simulink model "gm_hybrid_lht"  (R2019b)
settings: Solver=FixedStepDiscrete  StartTime=0.0  StopTime=inf  FixedStep=1/120e6  RelTol=1e-3
undefined symbols (not defined in the file or in its folder): bt, height, nTheta, width
libraries: hdlsllib x612, simulink x494, hdlmdlgenlib x7, dspsrcs4 x1
(part 2 of 17)

== system gm_hybrid_lht/Hybrid LHT/Hybrid LHT Kernel/Extract Active Votes ==
  note: Check the indices to ensure they are in the correct limits
  Theta : Inport  OutDataTypeStr=uint8  PortDimensions=1  SampleTime=8.33333333333333e-09
  Add : Sum  AccumDataTypeStr=fixdt(1, 10, 0)  OutDataTypeStr=fixdt(1, 10, 0)  SampleTime=8.33333333333333e-09
  Add1 : Sum  Inputs=+-  AccumDataTypeStr=fixdt(1, 12, 0)  OutDataTypeStr=fixdt(1, 12, 0)  SampleTime=8.33333333333333e-09
  Add2 : Sum  Inputs=+-  AccumDataTypeStr=fixdt(1, 9, 0)  OutDataTypeStr=fixdt(1, 9, 0)  SampleTime=8.33333333333333e-09
  Add3 : Sum  AccumDataTypeStr=fixdt(1, 11, 0)  OutDataTypeStr=fixdt(1, 11, 0)  SampleTime=8.33333333333333e-09
  Add4 : Sum  Inputs=+-  AccumDataTypeStr=uint8  OutDataTypeStr=uint8  SampleTime=8.33333333333333e-09
  Constant : Constant  Value=[-30 -29 -28 -27 -26 -25 -24 -23 -22 -21 -20 -19 -18 -17 -16 -15 -14 -13 -12 -11 -10 -9 -8 -7 -6 -5 -4 -3 -2 -1 0 1 2 3 4 5 6 7 8 9 10 11 12 13 14 15 16 17 18 19 20 21 22 23 24 25 26 27 28 29]  VectorParams1D=off  OutDataTypeStr=fixdt(1, 6, 0)  SampleTime=-1
  Data Type Conversion : DataTypeConversion  OutDataTypeStr=uint8  SampleTime=8.33333333333333e-09
  Data Type Conversion1 : DataTypeConversion  OutDataTypeStr=uint8  SampleTime=8.33333333333333e-09
  Gain1 : Product  Inputs=**  OutDataTypeStr=uint8  SampleTime=8.33333333333333e-09
  Gain1_const : Constant  Value=60  OutDataTypeStr=uint8  SampleTime=-1
  GetShift : Subsystem
  High : Constant  Value=59  OutDataTypeStr=uint8  SampleTime=-1
  High1 : Constant  Value=59  OutDataTypeStr=uint8  SampleTime=-1
  Low : Constant  Value=0  OutDataTypeStr=fixdt(0, 1, 0)  SampleTime=-1
  Multiport Switch2 : MultiPortSwitch  DataPortOrder=Zero-based contiguous  Inputs=2  DiagnosticForDefault=None  zeroidx=on  OutDataTypeStr=fixdt(1, 11, 0)  SampleTime=8.33333333333333e-09
  Multiport Switch3 : MultiPortSwitch  DataPortOrder=Zero-based contiguous  Inputs=2  DiagnosticForDefault=None  zeroidx=on  OutDataTypeStr=fixdt(1, 12, 0)  SampleTime=8.33333333333333e-09
  PipelineRegister : Delay  DelayLength=double(1)  InitialCondition=0  SampleTime=8.33333333333333e-09
  Relational : RelationalOperator  Operator=<  OutDataTypeStr=boolean  SampleTime=8.33333333333333e-09  RndMeth=Nearest
  Relational1 : RelationalOperator  Operator=>  OutDataTypeStr=boolean  SampleTime=8.33333333333333e-09  RndMeth=Nearest
  Selector4 : Selector  NumberOfDimensions=2  IndexMode=Zero-based  SampleTime=8.33333333333333e-09  IndexOptions=Index vector (dialog),Index vector (dialog)  Indices=double(0),double([59 58 57 56 55 54 53 52 51 50 49 48 47 46 45 44 43 42 41 40 39 38 37 36 35 34 33 32 31 30 29 28 27 26 25 24 23 22 21 20 19 18 17 16 15 14 13 12 11 10 9 8 7 6 5 4 3 2 1 0])  OutputSizes=double(1),double(1)
  delayMatch : Delay  DelayLength=double(1)  InitialCondition=0  SampleTime=8.33333333333333e-09
  nTheta : Constant  Value=60  OutDataTypeStr=uint8  SampleTime=-1
  Index : Outport  VectorParamsAs1DForOutWhenUnconnected=off
  wires:
  delayMatch/1 -> Add2/1
  Add/1 -> Relational/1, Multiport Switch2/2, Add3/1
  Add1/1 -> Multiport Switch3/3
  Add2/1 -> Add/1
  Add3/1 -> Multiport Switch2/3
  Add4/1 -> Selector4/1
  Constant/1 -> Add/2
  Data Type Conversion/1 -> Data Type Conversion1/1
  Data Type Conversion1/1 -> Add4/2
  PipelineRegister/1 -> Add2/2
  GetShift/1(Shift) -> Gain1/2
  High/1 -> Relational1/2
  High1/1 -> Add4/1
  Low/1 -> Relational/2
  Multiport Switch2/1 -> Relational1/1, Multiport Switch3/2, Add1/1
  Multiport Switch3/1 -> Data Type Conversion/1
  Relational/1 -> Multiport Switch2/1
  Relational1/1 -> Multiport Switch3/1
  Selector4/1 -> Index/1
  nTheta/1 -> Add3/2, Add1/2
  Gain1_const/1 -> Gain1/1
  Theta/1 -> delayMatch/1, GetShift/1(Theta)
  Gain1/1 -> PipelineRegister/1

== system gm_hybrid_lht/Hybrid LHT/Hybrid LHT Kernel/Gradient Kernel System ==
  Edge : Inport  OutDataTypeStr=fixdt(0, 1, 0)  PortDimensions=1  SampleTime=8.33333333333333e-09
  X : Inport  Port=2  OutDataTypeStr=fixdt(1, 10, 0)  PortDimensions=1  SampleTime=8.33333333333333e-09
  Y : Inport  Port=3  OutDataTypeStr=fixdt(1, 10, 0)  PortDimensions=1  SampleTime=8.33333333333333e-09
  Theta : Inport  Port=4  OutDataTypeStr=uint8  PortDimensions=1  SampleTime=8.33333333333333e-09
  Get Index and Fix Limits : Subsystem
  Hough Kernel : Subsystem
  vEdge : Outport  VectorParamsAs1DForOutWhenUnconnected=off
  Rho : Outport  Port=2  VectorParamsAs1DForOutWhenUnconnected=off
  Shift : Outport  Port=3  VectorParamsAs1DForOutWhenUnconnected=off
  wires:
  Get Index and Fix Limits/1(Index) -> Hough Kernel/4(Index)
  Get Index and Fix Limits/2(Shift) -> Shift/1
  Hough Kernel/1(vEdge) -> vEdge/1
  Hough Kernel/2(Rho) -> Rho/1
  Edge/1 -> Hough Kernel/1(Edge)
  X/1 -> Hough Kernel/2(X)
  Y/1 -> Hough Kernel/3(Y)
  Theta/1 -> Get Index and Fix Limits/1(Theta)

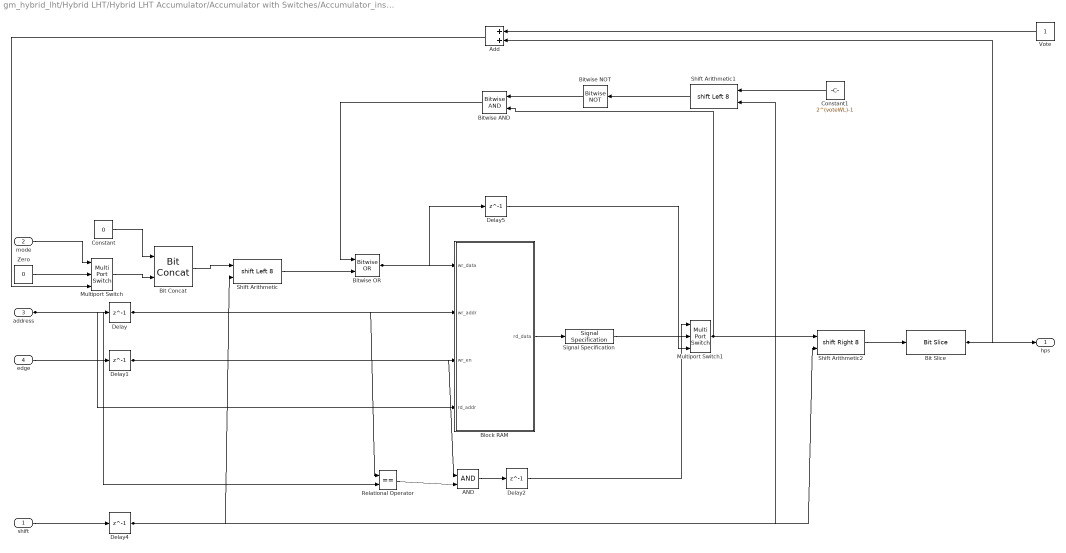
== system gm_hybrid_lht/Hybrid LHT/Hybrid LHT Accumulator/Accumulator with Switches/Accumulator_instance1 ==
  shift : Inport  OutDataTypeStr=fixdt(0, 6, 0)  PortDimensions=1  SampleTime=8.33333333333333e-09
  mode : Inport  Port=2  OutDataTypeStr=boolean  PortDimensions=1  SampleTime=8.33333333333333e-09
  address : Inport  Port=3  OutDataTypeStr=fixdt(0, 11, 0)  PortDimensions=1  SampleTime=8.33333333333333e-09
  edge : Inport  Port=4  OutDataTypeStr=boolean  PortDimensions=1  SampleTime=8.33333333333333e-09
  AND : Logic  IconShape=distinctive  AllPortsSameDT=off  OutDataTypeStr=boolean
  Add : Sum  OutDataTypeStr=fixdt(0, ceil(log2(maxRho*2)), 0)
  Bit Concat : hdlsllib/Logic and Bit Operations/Bit Concat  numInputs=2
      settings: SourceProductName=Simulink
  Bit Slice : hdlsllib/Logic and Bit Operations/Bit Slice  lidx=voteWL-1  ridx=0
  Bitwise AND : simulink/Logic and Bit Operations/Bitwise Operator  logicop=AND  UseBitMask=off  NumInputPorts=2  BitMask=bin2dec('11011001')  BitMaskRealWorld=Stored Integer
  Bitwise NOT : simulink/Logic and Bit Operations/Bitwise Operator  logicop=NOT  UseBitMask=off  BitMask=bin2dec('11011001')  BitMaskRealWorld=Stored Integer
  Bitwise OR : simulink/Logic and Bit Operations/Bitwise Operator  logicop=OR  UseBitMask=off  NumInputPorts=2  BitMask=bin2dec('11011001')  BitMaskRealWorld=Stored Integer
  Block RAM : Subsystem
  Constant : Constant  Value=0  OutDataTypeStr=fixdt(0, 36-voteWL, 0)  SampleTime=-1
  Constant1 : Constant  Value=2^(voteWL)-1  OutDataTypeStr=fixdt(0, 36, 0)  SampleTime=-1
  Delay{,1..2,4..5} (5 alike) : Delay  DelayLength=1
  Multiport Switch : MultiPortSwitch  DataPortOrder=Zero-based contiguous  Inputs=2  zeroidx=on
  Multiport Switch1 : MultiPortSwitch  DataPortOrder=Zero-based contiguous  Inputs=2  zeroidx=on
  Relational Operator : RelationalOperator  Operator===  OutDataTypeStr=boolean  RndMeth=Simplest
  Shift Arithmetic : ArithShift  BitShiftNumberSource=Input port  BitShiftNumber=8  BitShiftDirection=Left  DiagnosticForOORShift=Error
      settings: InputPortMap=u0,p1
  Shift Arithmetic1 : ArithShift  BitShiftNumberSource=Input port  BitShiftNumber=8  BitShiftDirection=Left  DiagnosticForOORShift=Error
      settings: InputPortMap=u0,p1
  Shift Arithmetic2 : ArithShift  BitShiftNumberSource=Input port  BitShiftNumber=8  BitShiftDirection=Right  DiagnosticForOORShift=Error
      settings: InputPortMap=u0,p1
  Signal Specification : SignalSpecification  OutDataTypeStr=fixdt(0, 36, 0)
  Vote : Constant  OutDataTypeStr=fixdt(0,1,0)  SampleTime=-1
  Zero : Constant  Value=0  OutDataTypeStr=fixdt(0,1,0)  SampleTime=-1
  hps : Outport
  wires:
  Zero/1 -> Multiport Switch/2
  Vote/1 -> Add/1
  Shift Arithmetic1/1 -> Bitwise NOT/1
  Relational Operator/1 -> AND/2
  Delay4/1 -> Shift Arithmetic1/2, Shift Arithmetic/2, Shift Arithmetic2/2
  Delay2/1 -> Multiport Switch1/1
  Delay1/1 -> AND/1, Block RAM/3(wr_en)
  Delay/1 -> Relational Operator/1, Block RAM/2(wr_addr)
  Constant1/1 -> Shift Arithmetic1/1
  Constant/1 -> Bit Concat/1
  Bitwise NOT/1 -> Bitwise AND/1
  Bit Slice/1 -> hps/1, Add/2
  AND/1 -> Delay2/1
  shift/1 -> Delay4/1
  mode/1 -> Multiport Switch/1
  address/1 -> Relational Operator/2, Delay/1, Block RAM/4(rd_addr)
  edge/1 -> Delay1/1
  Delay5/1 -> Multiport Switch1/3
  Shift Arithmetic/1 -> Bitwise OR/2
  Bit Concat/1 -> Shift Arithmetic/1
  Multiport Switch/1 -> Bit Concat/2
  Add/1 -> Multiport Switch/3
  Shift Arithmetic2/1 -> Bit Slice/1
  Bitwise AND/1 -> Bitwise OR/1
  Bitwise OR/1 -> Delay5/1, Block RAM/1(wr_data)
  Signal Specification/1 -> Multiport Switch1/2
  Multiport Switch1/1 -> Bitwise AND/2, Shift Arithmetic2/1
  Block RAM/1(rd_data) -> Signal Specification/1

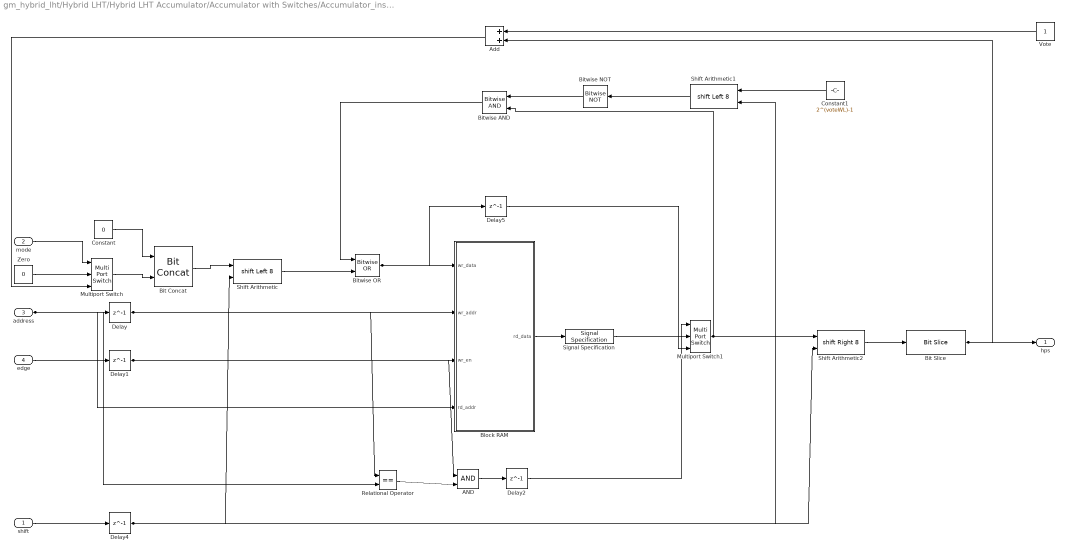
== system gm_hybrid_lht/Hybrid LHT/Hybrid LHT Accumulator/Accumulator with Switches/Accumulator_instance10 ==
  shift : Inport  OutDataTypeStr=fixdt(0, 6, 0)  PortDimensions=1  SampleTime=8.33333333333333e-09
  mode : Inport  Port=2  OutDataTypeStr=boolean  PortDimensions=1  SampleTime=8.33333333333333e-09
  address : Inport  Port=3  OutDataTypeStr=fixdt(0, 11, 0)  PortDimensions=1  SampleTime=8.33333333333333e-09
  edge : Inport  Port=4  OutDataTypeStr=boolean  PortDimensions=1  SampleTime=8.33333333333333e-09
  AND : Logic  IconShape=distinctive  AllPortsSameDT=off  OutDataTypeStr=boolean
  Add : Sum  OutDataTypeStr=fixdt(0, ceil(log2(maxRho*2)), 0)
  Bit Concat : hdlsllib/Logic and Bit Operations/Bit Concat  numInputs=2
      settings: SourceProductName=Simulink
  Bit Slice : hdlsllib/Logic and Bit Operations/Bit Slice  lidx=voteWL-1  ridx=0
  Bitwise AND : simulink/Logic and Bit Operations/Bitwise Operator  logicop=AND  UseBitMask=off  NumInputPorts=2  BitMask=bin2dec('11011001')  BitMaskRealWorld=Stored Integer
  Bitwise NOT : simulink/Logic and Bit Operations/Bitwise Operator  logicop=NOT  UseBitMask=off  BitMask=bin2dec('11011001')  BitMaskRealWorld=Stored Integer
  Bitwise OR : simulink/Logic and Bit Operations/Bitwise Operator  logicop=OR  UseBitMask=off  NumInputPorts=2  BitMask=bin2dec('11011001')  BitMaskRealWorld=Stored Integer
  Block RAM : Subsystem
  Constant : Constant  Value=0  OutDataTypeStr=fixdt(0, 36-voteWL, 0)  SampleTime=-1
  Constant1 : Constant  Value=2^(voteWL)-1  OutDataTypeStr=fixdt(0, 36, 0)  SampleTime=-1
  Delay{,1..2,4..5} (5 alike) : Delay  DelayLength=1
  Multiport Switch : MultiPortSwitch  DataPortOrder=Zero-based contiguous  Inputs=2  zeroidx=on
  Multiport Switch1 : MultiPortSwitch  DataPortOrder=Zero-based contiguous  Inputs=2  zeroidx=on
  Relational Operator : RelationalOperator  Operator===  OutDataTypeStr=boolean  RndMeth=Simplest
  Shift Arithmetic : ArithShift  BitShiftNumberSource=Input port  BitShiftNumber=8  BitShiftDirection=Left  DiagnosticForOORShift=Error
      settings: InputPortMap=u0,p1
  Shift Arithmetic1 : ArithShift  BitShiftNumberSource=Input port  BitShiftNumber=8  BitShiftDirection=Left  DiagnosticForOORShift=Error
      settings: InputPortMap=u0,p1
  Shift Arithmetic2 : ArithShift  BitShiftNumberSource=Input port  BitShiftNumber=8  BitShiftDirection=Right  DiagnosticForOORShift=Error
      settings: InputPortMap=u0,p1
  Signal Specification : SignalSpecification  OutDataTypeStr=fixdt(0, 36, 0)
  Vote : Constant  OutDataTypeStr=fixdt(0,1,0)  SampleTime=-1
  Zero : Constant  Value=0  OutDataTypeStr=fixdt(0,1,0)  SampleTime=-1
  hps : Outport
  wires:
  Block RAM/1(rd_data) -> Signal Specification/1
  Multiport Switch1/1 -> Shift Arithmetic2/1, Bitwise AND/2
  Signal Specification/1 -> Multiport Switch1/2
  Bitwise OR/1 -> Block RAM/1(wr_data), Delay5/1
  Bitwise AND/1 -> Bitwise OR/1
  Shift Arithmetic2/1 -> Bit Slice/1
  Add/1 -> Multiport Switch/3
  Multiport Switch/1 -> Bit Concat/2
  Bit Concat/1 -> Shift Arithmetic/1
  Shift Arithmetic/1 -> Bitwise OR/2
  Delay5/1 -> Multiport Switch1/3
  edge/1 -> Delay1/1
  address/1 -> Block RAM/4(rd_addr), Delay/1, Relational Operator/2
  mode/1 -> Multiport Switch/1
  shift/1 -> Delay4/1
  AND/1 -> Delay2/1
  Bit Slice/1 -> Add/2, hps/1
  Bitwise NOT/1 -> Bitwise AND/1
  Constant/1 -> Bit Concat/1
  Constant1/1 -> Shift Arithmetic1/1
  Delay/1 -> Block RAM/2(wr_addr), Relational Operator/1
  Delay1/1 -> Block RAM/3(wr_en), AND/1
  Delay2/1 -> Multiport Switch1/1
  Delay4/1 -> Shift Arithmetic2/2, Shift Arithmetic/2, Shift Arithmetic1/2
  Relational Operator/1 -> AND/2
  Shift Arithmetic1/1 -> Bitwise NOT/1
  Vote/1 -> Add/1
  Zero/1 -> Multiport Switch/2

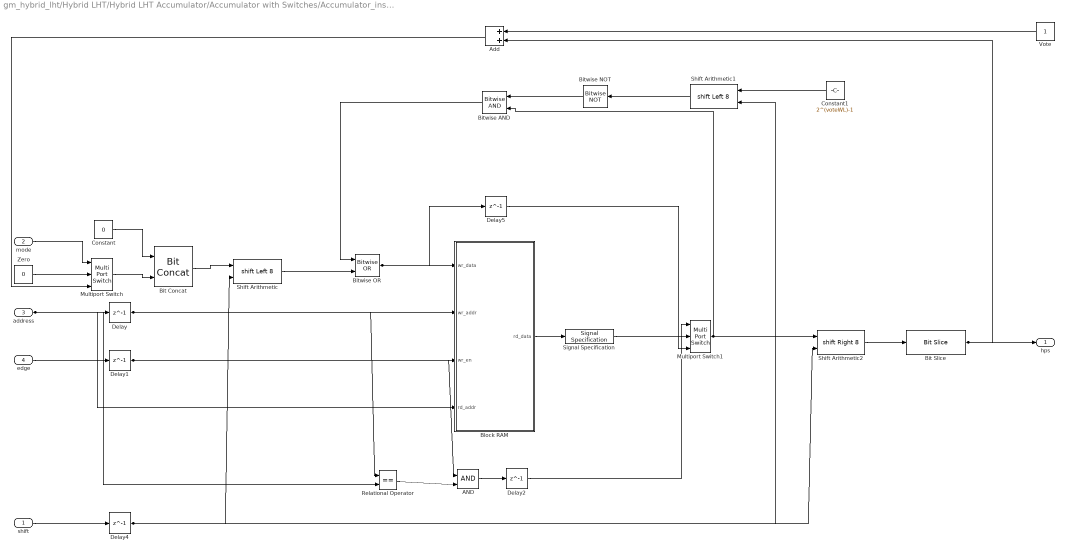
== system gm_hybrid_lht/Hybrid LHT/Hybrid LHT Accumulator/Accumulator with Switches/Accumulator_instance11 ==
  shift : Inport  OutDataTypeStr=fixdt(0, 6, 0)  PortDimensions=1  SampleTime=8.33333333333333e-09
  mode : Inport  Port=2  OutDataTypeStr=boolean  PortDimensions=1  SampleTime=8.33333333333333e-09
  address : Inport  Port=3  OutDataTypeStr=fixdt(0, 11, 0)  PortDimensions=1  SampleTime=8.33333333333333e-09
  edge : Inport  Port=4  OutDataTypeStr=boolean  PortDimensions=1  SampleTime=8.33333333333333e-09
  AND : Logic  IconShape=distinctive  AllPortsSameDT=off  OutDataTypeStr=boolean
  Add : Sum  OutDataTypeStr=fixdt(0, ceil(log2(maxRho*2)), 0)
  Bit Concat : hdlsllib/Logic and Bit Operations/Bit Concat  numInputs=2
      settings: SourceProductName=Simulink
  Bit Slice : hdlsllib/Logic and Bit Operations/Bit Slice  lidx=voteWL-1  ridx=0
  Bitwise AND : simulink/Logic and Bit Operations/Bitwise Operator  logicop=AND  UseBitMask=off  NumInputPorts=2  BitMask=bin2dec('11011001')  BitMaskRealWorld=Stored Integer
  Bitwise NOT : simulink/Logic and Bit Operations/Bitwise Operator  logicop=NOT  UseBitMask=off  BitMask=bin2dec('11011001')  BitMaskRealWorld=Stored Integer
  Bitwise OR : simulink/Logic and Bit Operations/Bitwise Operator  logicop=OR  UseBitMask=off  NumInputPorts=2  BitMask=bin2dec('11011001')  BitMaskRealWorld=Stored Integer
  Block RAM : Subsystem
  Constant : Constant  Value=0  OutDataTypeStr=fixdt(0, 36-voteWL, 0)  SampleTime=-1
  Constant1 : Constant  Value=2^(voteWL)-1  OutDataTypeStr=fixdt(0, 36, 0)  SampleTime=-1
  Delay{,1..2,4..5} (5 alike) : Delay  DelayLength=1
  Multiport Switch : MultiPortSwitch  DataPortOrder=Zero-based contiguous  Inputs=2  zeroidx=on
  Multiport Switch1 : MultiPortSwitch  DataPortOrder=Zero-based contiguous  Inputs=2  zeroidx=on
  Relational Operator : RelationalOperator  Operator===  OutDataTypeStr=boolean  RndMeth=Simplest
  Shift Arithmetic : ArithShift  BitShiftNumberSource=Input port  BitShiftNumber=8  BitShiftDirection=Left  DiagnosticForOORShift=Error
      settings: InputPortMap=u0,p1
  Shift Arithmetic1 : ArithShift  BitShiftNumberSource=Input port  BitShiftNumber=8  BitShiftDirection=Left  DiagnosticForOORShift=Error
      settings: InputPortMap=u0,p1
  Shift Arithmetic2 : ArithShift  BitShiftNumberSource=Input port  BitShiftNumber=8  BitShiftDirection=Right  DiagnosticForOORShift=Error
      settings: InputPortMap=u0,p1
  Signal Specification : SignalSpecification  OutDataTypeStr=fixdt(0, 36, 0)
  Vote : Constant  OutDataTypeStr=fixdt(0,1,0)  SampleTime=-1
  Zero : Constant  Value=0  OutDataTypeStr=fixdt(0,1,0)  SampleTime=-1
  hps : Outport
  wires:
  Block RAM/1(rd_data) -> Signal Specification/1
  Multiport Switch1/1 -> Shift Arithmetic2/1, Bitwise AND/2
  Signal Specification/1 -> Multiport Switch1/2
  Bitwise OR/1 -> Block RAM/1(wr_data), Delay5/1
  Bitwise AND/1 -> Bitwise OR/1
  Shift Arithmetic2/1 -> Bit Slice/1
  Add/1 -> Multiport Switch/3
  Multiport Switch/1 -> Bit Concat/2
  Bit Concat/1 -> Shift Arithmetic/1
  Shift Arithmetic/1 -> Bitwise OR/2
  Delay5/1 -> Multiport Switch1/3
  edge/1 -> Delay1/1
  address/1 -> Block RAM/4(rd_addr), Delay/1, Relational Operator/2
  mode/1 -> Multiport Switch/1
  shift/1 -> Delay4/1
  AND/1 -> Delay2/1
  Bit Slice/1 -> Add/2, hps/1
  Bitwise NOT/1 -> Bitwise AND/1
  Constant/1 -> Bit Concat/1
  Constant1/1 -> Shift Arithmetic1/1
  Delay/1 -> Block RAM/2(wr_addr), Relational Operator/1
  Delay1/1 -> Block RAM/3(wr_en), AND/1
  Delay2/1 -> Multiport Switch1/1
  Delay4/1 -> Shift Arithmetic2/2, Shift Arithmetic/2, Shift Arithmetic1/2
  Relational Operator/1 -> AND/2
  Shift Arithmetic1/1 -> Bitwise NOT/1
  Vote/1 -> Add/1
  Zero/1 -> Multiport Switch/2

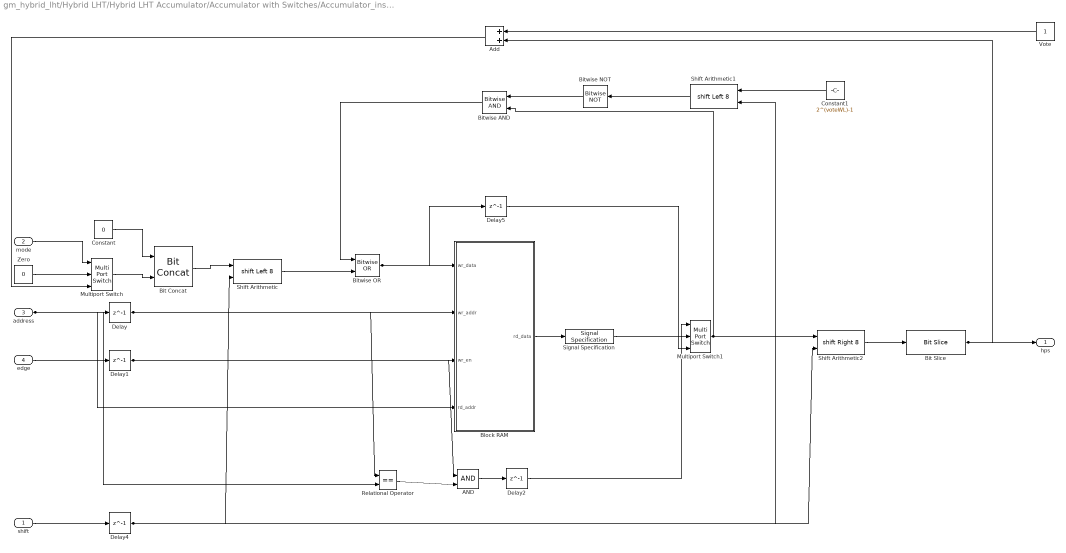
== system gm_hybrid_lht/Hybrid LHT/Hybrid LHT Accumulator/Accumulator with Switches/Accumulator_instance12 ==
  shift : Inport  OutDataTypeStr=fixdt(0, 6, 0)  PortDimensions=1  SampleTime=8.33333333333333e-09
  mode : Inport  Port=2  OutDataTypeStr=boolean  PortDimensions=1  SampleTime=8.33333333333333e-09
  address : Inport  Port=3  OutDataTypeStr=fixdt(0, 11, 0)  PortDimensions=1  SampleTime=8.33333333333333e-09
  edge : Inport  Port=4  OutDataTypeStr=boolean  PortDimensions=1  SampleTime=8.33333333333333e-09
  AND : Logic  IconShape=distinctive  AllPortsSameDT=off  OutDataTypeStr=boolean
  Add : Sum  OutDataTypeStr=fixdt(0, ceil(log2(maxRho*2)), 0)
  Bit Concat : hdlsllib/Logic and Bit Operations/Bit Concat  numInputs=2
      settings: SourceProductName=Simulink
  Bit Slice : hdlsllib/Logic and Bit Operations/Bit Slice  lidx=voteWL-1  ridx=0
  Bitwise AND : simulink/Logic and Bit Operations/Bitwise Operator  logicop=AND  UseBitMask=off  NumInputPorts=2  BitMask=bin2dec('11011001')  BitMaskRealWorld=Stored Integer
  Bitwise NOT : simulink/Logic and Bit Operations/Bitwise Operator  logicop=NOT  UseBitMask=off  BitMask=bin2dec('11011001')  BitMaskRealWorld=Stored Integer
  Bitwise OR : simulink/Logic and Bit Operations/Bitwise Operator  logicop=OR  UseBitMask=off  NumInputPorts=2  BitMask=bin2dec('11011001')  BitMaskRealWorld=Stored Integer
  Block RAM : Subsystem
  Constant : Constant  Value=0  OutDataTypeStr=fixdt(0, 36-voteWL, 0)  SampleTime=-1
  Constant1 : Constant  Value=2^(voteWL)-1  OutDataTypeStr=fixdt(0, 36, 0)  SampleTime=-1
  Delay{,1..2,4..5} (5 alike) : Delay  DelayLength=1
  Multiport Switch : MultiPortSwitch  DataPortOrder=Zero-based contiguous  Inputs=2  zeroidx=on
  Multiport Switch1 : MultiPortSwitch  DataPortOrder=Zero-based contiguous  Inputs=2  zeroidx=on
  Relational Operator : RelationalOperator  Operator===  OutDataTypeStr=boolean  RndMeth=Simplest
  Shift Arithmetic : ArithShift  BitShiftNumberSource=Input port  BitShiftNumber=8  BitShiftDirection=Left  DiagnosticForOORShift=Error
      settings: InputPortMap=u0,p1
  Shift Arithmetic1 : ArithShift  BitShiftNumberSource=Input port  BitShiftNumber=8  BitShiftDirection=Left  DiagnosticForOORShift=Error
      settings: InputPortMap=u0,p1
  Shift Arithmetic2 : ArithShift  BitShiftNumberSource=Input port  BitShiftNumber=8  BitShiftDirection=Right  DiagnosticForOORShift=Error
      settings: InputPortMap=u0,p1
  Signal Specification : SignalSpecification  OutDataTypeStr=fixdt(0, 36, 0)
  Vote : Constant  OutDataTypeStr=fixdt(0,1,0)  SampleTime=-1
  Zero : Constant  Value=0  OutDataTypeStr=fixdt(0,1,0)  SampleTime=-1
  hps : Outport
  wires:
  Block RAM/1(rd_data) -> Signal Specification/1
  Multiport Switch1/1 -> Shift Arithmetic2/1, Bitwise AND/2
  Signal Specification/1 -> Multiport Switch1/2
  Bitwise OR/1 -> Block RAM/1(wr_data), Delay5/1
  Bitwise AND/1 -> Bitwise OR/1
  Shift Arithmetic2/1 -> Bit Slice/1
  Add/1 -> Multiport Switch/3
  Multiport Switch/1 -> Bit Concat/2
  Bit Concat/1 -> Shift Arithmetic/1
  Shift Arithmetic/1 -> Bitwise OR/2
  Delay5/1 -> Multiport Switch1/3
  edge/1 -> Delay1/1
  address/1 -> Block RAM/4(rd_addr), Delay/1, Relational Operator/2
  mode/1 -> Multiport Switch/1
  shift/1 -> Delay4/1
  AND/1 -> Delay2/1
  Bit Slice/1 -> Add/2, hps/1
  Bitwise NOT/1 -> Bitwise AND/1
  Constant/1 -> Bit Concat/1
  Constant1/1 -> Shift Arithmetic1/1
  Delay/1 -> Block RAM/2(wr_addr), Relational Operator/1
  Delay1/1 -> Block RAM/3(wr_en), AND/1
  Delay2/1 -> Multiport Switch1/1
  Delay4/1 -> Shift Arithmetic2/2, Shift Arithmetic/2, Shift Arithmetic1/2
  Relational Operator/1 -> AND/2
  Shift Arithmetic1/1 -> Bitwise NOT/1
  Vote/1 -> Add/1
  Zero/1 -> Multiport Switch/2

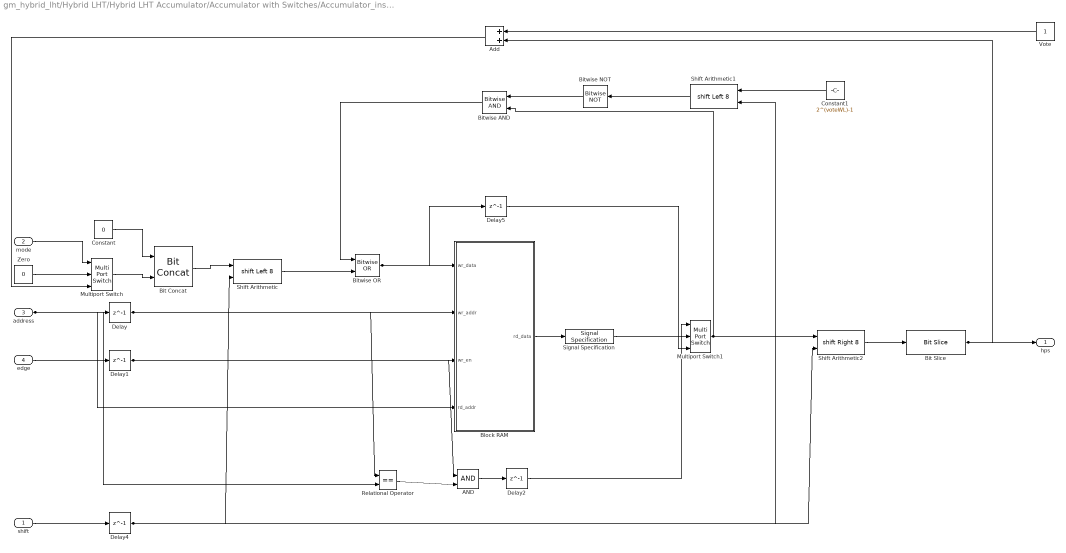
== system gm_hybrid_lht/Hybrid LHT/Hybrid LHT Accumulator/Accumulator with Switches/Accumulator_instance13 ==
  shift : Inport  OutDataTypeStr=fixdt(0, 6, 0)  PortDimensions=1  SampleTime=8.33333333333333e-09
  mode : Inport  Port=2  OutDataTypeStr=boolean  PortDimensions=1  SampleTime=8.33333333333333e-09
  address : Inport  Port=3  OutDataTypeStr=fixdt(0, 11, 0)  PortDimensions=1  SampleTime=8.33333333333333e-09
  edge : Inport  Port=4  OutDataTypeStr=boolean  PortDimensions=1  SampleTime=8.33333333333333e-09
  AND : Logic  IconShape=distinctive  AllPortsSameDT=off  OutDataTypeStr=boolean
  Add : Sum  OutDataTypeStr=fixdt(0, ceil(log2(maxRho*2)), 0)
  Bit Concat : hdlsllib/Logic and Bit Operations/Bit Concat  numInputs=2
      settings: SourceProductName=Simulink
  Bit Slice : hdlsllib/Logic and Bit Operations/Bit Slice  lidx=voteWL-1  ridx=0
  Bitwise AND : simulink/Logic and Bit Operations/Bitwise Operator  logicop=AND  UseBitMask=off  NumInputPorts=2  BitMask=bin2dec('11011001')  BitMaskRealWorld=Stored Integer
  Bitwise NOT : simulink/Logic and Bit Operations/Bitwise Operator  logicop=NOT  UseBitMask=off  BitMask=bin2dec('11011001')  BitMaskRealWorld=Stored Integer
  Bitwise OR : simulink/Logic and Bit Operations/Bitwise Operator  logicop=OR  UseBitMask=off  NumInputPorts=2  BitMask=bin2dec('11011001')  BitMaskRealWorld=Stored Integer
  Block RAM : Subsystem
  Constant : Constant  Value=0  OutDataTypeStr=fixdt(0, 36-voteWL, 0)  SampleTime=-1
  Constant1 : Constant  Value=2^(voteWL)-1  OutDataTypeStr=fixdt(0, 36, 0)  SampleTime=-1
  Delay{,1..2,4..5} (5 alike) : Delay  DelayLength=1
  Multiport Switch : MultiPortSwitch  DataPortOrder=Zero-based contiguous  Inputs=2  zeroidx=on
  Multiport Switch1 : MultiPortSwitch  DataPortOrder=Zero-based contiguous  Inputs=2  zeroidx=on
  Relational Operator : RelationalOperator  Operator===  OutDataTypeStr=boolean  RndMeth=Simplest
  Shift Arithmetic : ArithShift  BitShiftNumberSource=Input port  BitShiftNumber=8  BitShiftDirection=Left  DiagnosticForOORShift=Error
      settings: InputPortMap=u0,p1
  Shift Arithmetic1 : ArithShift  BitShiftNumberSource=Input port  BitShiftNumber=8  BitShiftDirection=Left  DiagnosticForOORShift=Error
      settings: InputPortMap=u0,p1
  Shift Arithmetic2 : ArithShift  BitShiftNumberSource=Input port  BitShiftNumber=8  BitShiftDirection=Right  DiagnosticForOORShift=Error
      settings: InputPortMap=u0,p1
  Signal Specification : SignalSpecification  OutDataTypeStr=fixdt(0, 36, 0)
  Vote : Constant  OutDataTypeStr=fixdt(0,1,0)  SampleTime=-1
  Zero : Constant  Value=0  OutDataTypeStr=fixdt(0,1,0)  SampleTime=-1
  hps : Outport
  wires:
  Block RAM/1(rd_data) -> Signal Specification/1
  Multiport Switch1/1 -> Shift Arithmetic2/1, Bitwise AND/2
  Signal Specification/1 -> Multiport Switch1/2
  Bitwise OR/1 -> Block RAM/1(wr_data), Delay5/1
  Bitwise AND/1 -> Bitwise OR/1
  Shift Arithmetic2/1 -> Bit Slice/1
  Add/1 -> Multiport Switch/3
  Multiport Switch/1 -> Bit Concat/2
  Bit Concat/1 -> Shift Arithmetic/1
  Shift Arithmetic/1 -> Bitwise OR/2
  Delay5/1 -> Multiport Switch1/3
  edge/1 -> Delay1/1
  address/1 -> Block RAM/4(rd_addr), Delay/1, Relational Operator/2
  mode/1 -> Multiport Switch/1
  shift/1 -> Delay4/1
  AND/1 -> Delay2/1
  Bit Slice/1 -> Add/2, hps/1
  Bitwise NOT/1 -> Bitwise AND/1
  Constant/1 -> Bit Concat/1
  Constant1/1 -> Shift Arithmetic1/1
  Delay/1 -> Block RAM/2(wr_addr), Relational Operator/1
  Delay1/1 -> Block RAM/3(wr_en), AND/1
  Delay2/1 -> Multiport Switch1/1
  Delay4/1 -> Shift Arithmetic2/2, Shift Arithmetic/2, Shift Arithmetic1/2
  Relational Operator/1 -> AND/2
  Shift Arithmetic1/1 -> Bitwise NOT/1
  Vote/1 -> Add/1
  Zero/1 -> Multiport Switch/2

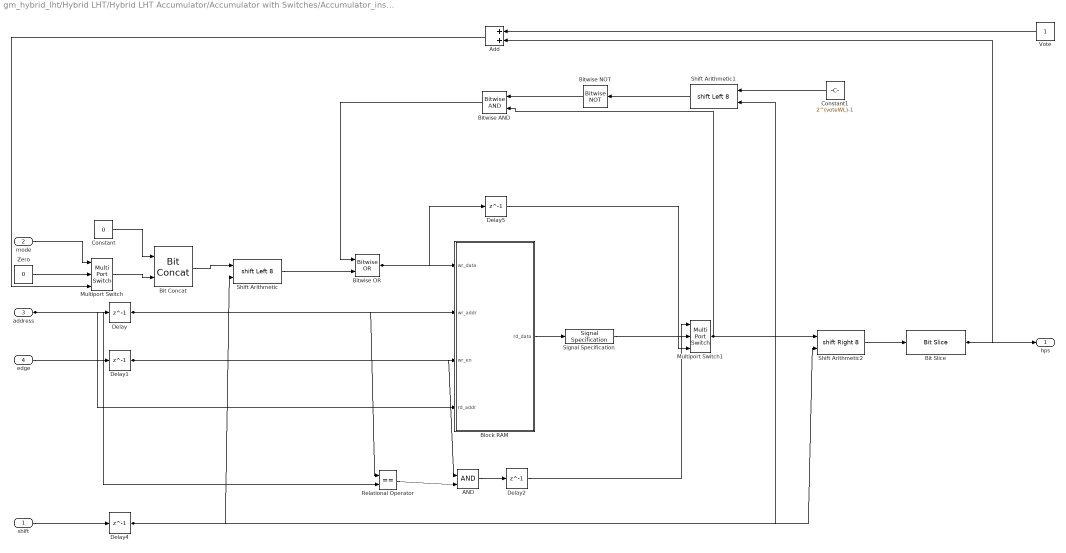
== system gm_hybrid_lht/Hybrid LHT/Hybrid LHT Accumulator/Accumulator with Switches/Accumulator_instance14 ==
  shift : Inport  OutDataTypeStr=fixdt(0, 6, 0)  PortDimensions=1  SampleTime=8.33333333333333e-09
  mode : Inport  Port=2  OutDataTypeStr=boolean  PortDimensions=1  SampleTime=8.33333333333333e-09
  address : Inport  Port=3  OutDataTypeStr=fixdt(0, 11, 0)  PortDimensions=1  SampleTime=8.33333333333333e-09
  edge : Inport  Port=4  OutDataTypeStr=boolean  PortDimensions=1  SampleTime=8.33333333333333e-09
  AND : Logic  IconShape=distinctive  AllPortsSameDT=off  OutDataTypeStr=boolean
  Add : Sum  OutDataTypeStr=fixdt(0, ceil(log2(maxRho*2)), 0)
  Bit Concat : hdlsllib/Logic and Bit Operations/Bit Concat  numInputs=2
      settings: SourceProductName=Simulink
  Bit Slice : hdlsllib/Logic and Bit Operations/Bit Slice  lidx=voteWL-1  ridx=0
  Bitwise AND : simulink/Logic and Bit Operations/Bitwise Operator  logicop=AND  UseBitMask=off  NumInputPorts=2  BitMask=bin2dec('11011001')  BitMaskRealWorld=Stored Integer
  Bitwise NOT : simulink/Logic and Bit Operations/Bitwise Operator  logicop=NOT  UseBitMask=off  BitMask=bin2dec('11011001')  BitMaskRealWorld=Stored Integer
  Bitwise OR : simulink/Logic and Bit Operations/Bitwise Operator  logicop=OR  UseBitMask=off  NumInputPorts=2  BitMask=bin2dec('11011001')  BitMaskRealWorld=Stored Integer
  Block RAM : Subsystem
  Constant : Constant  Value=0  OutDataTypeStr=fixdt(0, 36-voteWL, 0)  SampleTime=-1
  Constant1 : Constant  Value=2^(voteWL)-1  OutDataTypeStr=fixdt(0, 36, 0)  SampleTime=-1
  Delay{,1..2,4..5} (5 alike) : Delay  DelayLength=1
  Multiport Switch : MultiPortSwitch  DataPortOrder=Zero-based contiguous  Inputs=2  zeroidx=on
  Multiport Switch1 : MultiPortSwitch  DataPortOrder=Zero-based contiguous  Inputs=2  zeroidx=on
  Relational Operator : RelationalOperator  Operator===  OutDataTypeStr=boolean  RndMeth=Simplest
  Shift Arithmetic : ArithShift  BitShiftNumberSource=Input port  BitShiftNumber=8  BitShiftDirection=Left  DiagnosticForOORShift=Error
      settings: InputPortMap=u0,p1
  Shift Arithmetic1 : ArithShift  BitShiftNumberSource=Input port  BitShiftNumber=8  BitShiftDirection=Left  DiagnosticForOORShift=Error
      settings: InputPortMap=u0,p1
  Shift Arithmetic2 : ArithShift  BitShiftNumberSource=Input port  BitShiftNumber=8  BitShiftDirection=Right  DiagnosticForOORShift=Error
      settings: InputPortMap=u0,p1
  Signal Specification : SignalSpecification  OutDataTypeStr=fixdt(0, 36, 0)
  Vote : Constant  OutDataTypeStr=fixdt(0,1,0)  SampleTime=-1
  Zero : Constant  Value=0  OutDataTypeStr=fixdt(0,1,0)  SampleTime=-1
  hps : Outport
  wires:
  Block RAM/1(rd_data) -> Signal Specification/1
  Multiport Switch1/1 -> Shift Arithmetic2/1, Bitwise AND/2
  Signal Specification/1 -> Multiport Switch1/2
  Bitwise OR/1 -> Block RAM/1(wr_data), Delay5/1
  Bitwise AND/1 -> Bitwise OR/1
  Shift Arithmetic2/1 -> Bit Slice/1
  Add/1 -> Multiport Switch/3
  Multiport Switch/1 -> Bit Concat/2
  Bit Concat/1 -> Shift Arithmetic/1
  Shift Arithmetic/1 -> Bitwise OR/2
  Delay5/1 -> Multiport Switch1/3
  edge/1 -> Delay1/1
  address/1 -> Block RAM/4(rd_addr), Delay/1, Relational Operator/2
  mode/1 -> Multiport Switch/1
  shift/1 -> Delay4/1
  AND/1 -> Delay2/1
  Bit Slice/1 -> Add/2, hps/1
  Bitwise NOT/1 -> Bitwise AND/1
  Constant/1 -> Bit Concat/1
  Constant1/1 -> Shift Arithmetic1/1
  Delay/1 -> Block RAM/2(wr_addr), Relational Operator/1
  Delay1/1 -> Block RAM/3(wr_en), AND/1
  Delay2/1 -> Multiport Switch1/1
  Delay4/1 -> Shift Arithmetic2/2, Shift Arithmetic/2, Shift Arithmetic1/2
  Relational Operator/1 -> AND/2
  Shift Arithmetic1/1 -> Bitwise NOT/1
  Vote/1 -> Add/1
  Zero/1 -> Multiport Switch/2

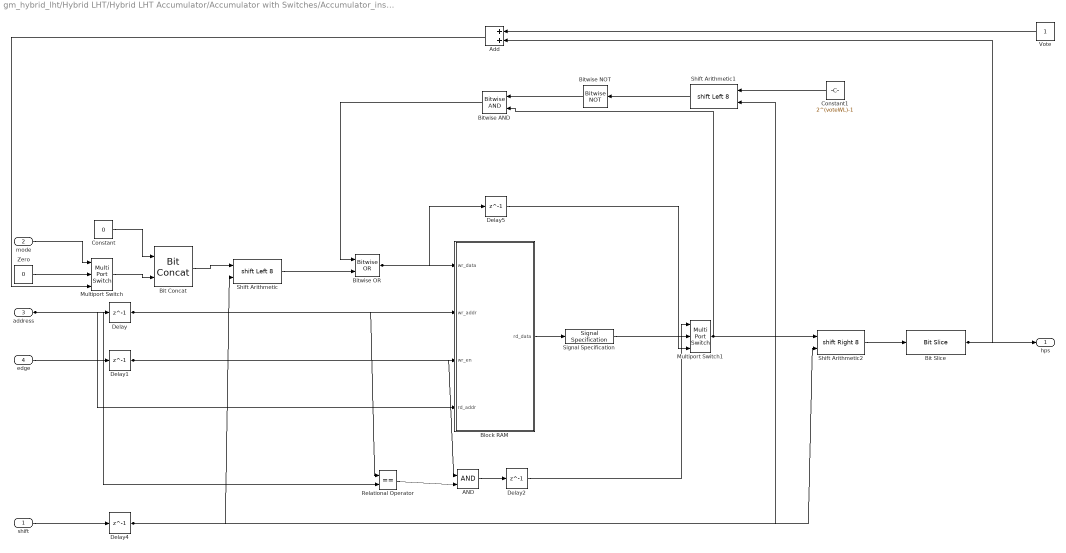
== system gm_hybrid_lht/Hybrid LHT/Hybrid LHT Accumulator/Accumulator with Switches/Accumulator_instance15 ==
  shift : Inport  OutDataTypeStr=fixdt(0, 6, 0)  PortDimensions=1  SampleTime=8.33333333333333e-09
  mode : Inport  Port=2  OutDataTypeStr=boolean  PortDimensions=1  SampleTime=8.33333333333333e-09
  address : Inport  Port=3  OutDataTypeStr=fixdt(0, 11, 0)  PortDimensions=1  SampleTime=8.33333333333333e-09
  edge : Inport  Port=4  OutDataTypeStr=boolean  PortDimensions=1  SampleTime=8.33333333333333e-09
  AND : Logic  IconShape=distinctive  AllPortsSameDT=off  OutDataTypeStr=boolean
  Add : Sum  OutDataTypeStr=fixdt(0, ceil(log2(maxRho*2)), 0)
  Bit Concat : hdlsllib/Logic and Bit Operations/Bit Concat  numInputs=2
      settings: SourceProductName=Simulink
  Bit Slice : hdlsllib/Logic and Bit Operations/Bit Slice  lidx=voteWL-1  ridx=0
  Bitwise AND : simulink/Logic and Bit Operations/Bitwise Operator  logicop=AND  UseBitMask=off  NumInputPorts=2  BitMask=bin2dec('11011001')  BitMaskRealWorld=Stored Integer
  Bitwise NOT : simulink/Logic and Bit Operations/Bitwise Operator  logicop=NOT  UseBitMask=off  BitMask=bin2dec('11011001')  BitMaskRealWorld=Stored Integer
  Bitwise OR : simulink/Logic and Bit Operations/Bitwise Operator  logicop=OR  UseBitMask=off  NumInputPorts=2  BitMask=bin2dec('11011001')  BitMaskRealWorld=Stored Integer
  Block RAM : Subsystem
  Constant : Constant  Value=0  OutDataTypeStr=fixdt(0, 36-voteWL, 0)  SampleTime=-1
  Constant1 : Constant  Value=2^(voteWL)-1  OutDataTypeStr=fixdt(0, 36, 0)  SampleTime=-1
  Delay{,1..2,4..5} (5 alike) : Delay  DelayLength=1
  Multiport Switch : MultiPortSwitch  DataPortOrder=Zero-based contiguous  Inputs=2  zeroidx=on
  Multiport Switch1 : MultiPortSwitch  DataPortOrder=Zero-based contiguous  Inputs=2  zeroidx=on
  Relational Operator : RelationalOperator  Operator===  OutDataTypeStr=boolean  RndMeth=Simplest
  Shift Arithmetic : ArithShift  BitShiftNumberSource=Input port  BitShiftNumber=8  BitShiftDirection=Left  DiagnosticForOORShift=Error
      settings: InputPortMap=u0,p1
  Shift Arithmetic1 : ArithShift  BitShiftNumberSource=Input port  BitShiftNumber=8  BitShiftDirection=Left  DiagnosticForOORShift=Error
      settings: InputPortMap=u0,p1
  Shift Arithmetic2 : ArithShift  BitShiftNumberSource=Input port  BitShiftNumber=8  BitShiftDirection=Right  DiagnosticForOORShift=Error
      settings: InputPortMap=u0,p1
  Signal Specification : SignalSpecification  OutDataTypeStr=fixdt(0, 36, 0)
  Vote : Constant  OutDataTypeStr=fixdt(0,1,0)  SampleTime=-1
  Zero : Constant  Value=0  OutDataTypeStr=fixdt(0,1,0)  SampleTime=-1
  hps : Outport
  wires:
  Block RAM/1(rd_data) -> Signal Specification/1
  Multiport Switch1/1 -> Shift Arithmetic2/1, Bitwise AND/2
  Signal Specification/1 -> Multiport Switch1/2
  Bitwise OR/1 -> Block RAM/1(wr_data), Delay5/1
  Bitwise AND/1 -> Bitwise OR/1
  Shift Arithmetic2/1 -> Bit Slice/1
  Add/1 -> Multiport Switch/3
  Multiport Switch/1 -> Bit Concat/2
  Bit Concat/1 -> Shift Arithmetic/1
  Shift Arithmetic/1 -> Bitwise OR/2
  Delay5/1 -> Multiport Switch1/3
  edge/1 -> Delay1/1
  address/1 -> Block RAM/4(rd_addr), Delay/1, Relational Operator/2
  mode/1 -> Multiport Switch/1
  shift/1 -> Delay4/1
  AND/1 -> Delay2/1
  Bit Slice/1 -> Add/2, hps/1
  Bitwise NOT/1 -> Bitwise AND/1
  Constant/1 -> Bit Concat/1
  Constant1/1 -> Shift Arithmetic1/1
  Delay/1 -> Block RAM/2(wr_addr), Relational Operator/1
  Delay1/1 -> Block RAM/3(wr_en), AND/1
  Delay2/1 -> Multiport Switch1/1
  Delay4/1 -> Shift Arithmetic2/2, Shift Arithmetic/2, Shift Arithmetic1/2
  Relational Operator/1 -> AND/2
  Shift Arithmetic1/1 -> Bitwise NOT/1
  Vote/1 -> Add/1
  Zero/1 -> Multiport Switch/2

== system gm_hybrid_lht/Hybrid LHT/Hybrid LHT Accumulator/Accumulator with Switches/Accumulator_instance16 ==
  shift : Inport  OutDataTypeStr=fixdt(0, 6, 0)  PortDimensions=1  SampleTime=8.33333333333333e-09
  mode : Inport  Port=2  OutDataTypeStr=boolean  PortDimensions=1  SampleTime=8.33333333333333e-09
  address : Inport  Port=3  OutDataTypeStr=fixdt(0, 11, 0)  PortDimensions=1  SampleTime=8.33333333333333e-09
  edge : Inport  Port=4  OutDataTypeStr=boolean  PortDimensions=1  SampleTime=8.33333333333333e-09
  AND : Logic  IconShape=distinctive  AllPortsSameDT=off  OutDataTypeStr=boolean
  Add : Sum  OutDataTypeStr=fixdt(0, ceil(log2(maxRho*2)), 0)
  Bit Concat : hdlsllib/Logic and Bit Operations/Bit Concat  numInputs=2
      settings: SourceProductName=Simulink
  Bit Slice : hdlsllib/Logic and Bit Operations/Bit Slice  lidx=voteWL-1  ridx=0
  Bitwise AND : simulink/Logic and Bit Operations/Bitwise Operator  logicop=AND  UseBitMask=off  NumInputPorts=2  BitMask=bin2dec('11011001')  BitMaskRealWorld=Stored Integer
  Bitwise NOT : simulink/Logic and Bit Operations/Bitwise Operator  logicop=NOT  UseBitMask=off  BitMask=bin2dec('11011001')  BitMaskRealWorld=Stored Integer
  Bitwise OR : simulink/Logic and Bit Operations/Bitwise Operator  logicop=OR  UseBitMask=off  NumInputPorts=2  BitMask=bin2dec('11011001')  BitMaskRealWorld=Stored Integer
  Block RAM : Subsystem
  Constant : Constant  Value=0  OutDataTypeStr=fixdt(0, 36-voteWL, 0)  SampleTime=-1
  Constant1 : Constant  Value=2^(voteWL)-1  OutDataTypeStr=fixdt(0, 36, 0)  SampleTime=-1
  Delay{,1..2,4..5} (5 alike) : Delay  DelayLength=1
  Multiport Switch : MultiPortSwitch  DataPortOrder=Zero-based contiguous  Inputs=2  zeroidx=on
  Multiport Switch1 : MultiPortSwitch  DataPortOrder=Zero-based contiguous  Inputs=2  zeroidx=on
  Relational Operator : RelationalOperator  Operator===  OutDataTypeStr=boolean  RndMeth=Simplest
  Shift Arithmetic : ArithShift  BitShiftNumberSource=Input port  BitShiftNumber=8  BitShiftDirection=Left  DiagnosticForOORShift=Error
      settings: InputPortMap=u0,p1
  Shift Arithmetic1 : ArithShift  BitShiftNumberSource=Input port  BitShiftNumber=8  BitShiftDirection=Left  DiagnosticForOORShift=Error
      settings: InputPortMap=u0,p1
  Shift Arithmetic2 : ArithShift  BitShiftNumberSource=Input port  BitShiftNumber=8  BitShiftDirection=Right  DiagnosticForOORShift=Error
      settings: InputPortMap=u0,p1
  Signal Specification : SignalSpecification  OutDataTypeStr=fixdt(0, 36, 0)
  Vote : Constant  OutDataTypeStr=fixdt(0,1,0)  SampleTime=-1
  Zero : Constant  Value=0  OutDataTypeStr=fixdt(0,1,0)  SampleTime=-1
  hps : Outport
  wires:
  Block RAM/1(rd_data) -> Signal Specification/1
  Multiport Switch1/1 -> Shift Arithmetic2/1, Bitwise AND/2
  Signal Specification/1 -> Multiport Switch1/2
  Bitwise OR/1 -> Block RAM/1(wr_data), Delay5/1
  Bitwise AND/1 -> Bitwise OR/1
  Shift Arithmetic2/1 -> Bit Slice/1
  Add/1 -> Multiport Switch/3
  Multiport Switch/1 -> Bit Concat/2
  Bit Concat/1 -> Shift Arithmetic/1
  Shift Arithmetic/1 -> Bitwise OR/2
  Delay5/1 -> Multiport Switch1/3
  edge/1 -> Delay1/1
  address/1 -> Block RAM/4(rd_addr), Delay/1, Relational Operator/2
  mode/1 -> Multiport Switch/1
  shift/1 -> Delay4/1
  AND/1 -> Delay2/1
  Bit Slice/1 -> Add/2, hps/1
  Bitwise NOT/1 -> Bitwise AND/1
  Constant/1 -> Bit Concat/1
  Constant1/1 -> Shift Arithmetic1/1
  Delay/1 -> Block RAM/2(wr_addr), Relational Operator/1
  Delay1/1 -> Block RAM/3(wr_en), AND/1
  Delay2/1 -> Multiport Switch1/1
  Delay4/1 -> Shift Arithmetic2/2, Shift Arithmetic/2, Shift Arithmetic1/2
  Relational Operator/1 -> AND/2
  Shift Arithmetic1/1 -> Bitwise NOT/1
  Vote/1 -> Add/1
  Zero/1 -> Multiport Switch/2

== system gm_hybrid_lht/Hybrid LHT/Hybrid LHT Accumulator/Accumulator with Switches/Accumulator_instance17 ==
  shift : Inport  OutDataTypeStr=fixdt(0, 6, 0)  PortDimensions=1  SampleTime=8.33333333333333e-09
  mode : Inport  Port=2  OutDataTypeStr=boolean  PortDimensions=1  SampleTime=8.33333333333333e-09
  address : Inport  Port=3  OutDataTypeStr=fixdt(0, 11, 0)  PortDimensions=1  SampleTime=8.33333333333333e-09
  edge : Inport  Port=4  OutDataTypeStr=boolean  PortDimensions=1  SampleTime=8.33333333333333e-09
  AND : Logic  IconShape=distinctive  AllPortsSameDT=off  OutDataTypeStr=boolean
  Add : Sum  OutDataTypeStr=fixdt(0, ceil(log2(maxRho*2)), 0)
  Bit Concat : hdlsllib/Logic and Bit Operations/Bit Concat  numInputs=2
      settings: SourceProductName=Simulink
  Bit Slice : hdlsllib/Logic and Bit Operations/Bit Slice  lidx=voteWL-1  ridx=0
  Bitwise AND : simulink/Logic and Bit Operations/Bitwise Operator  logicop=AND  UseBitMask=off  NumInputPorts=2  BitMask=bin2dec('11011001')  BitMaskRealWorld=Stored Integer
  Bitwise NOT : simulink/Logic and Bit Operations/Bitwise Operator  logicop=NOT  UseBitMask=off  BitMask=bin2dec('11011001')  BitMaskRealWorld=Stored Integer
  Bitwise OR : simulink/Logic and Bit Operations/Bitwise Operator  logicop=OR  UseBitMask=off  NumInputPorts=2  BitMask=bin2dec('11011001')  BitMaskRealWorld=Stored Integer
  Block RAM : Subsystem
  Constant : Constant  Value=0  OutDataTypeStr=fixdt(0, 36-voteWL, 0)  SampleTime=-1
  Constant1 : Constant  Value=2^(voteWL)-1  OutDataTypeStr=fixdt(0, 36, 0)  SampleTime=-1
  Delay{,1..2,4..5} (5 alike) : Delay  DelayLength=1
  Multiport Switch : MultiPortSwitch  DataPortOrder=Zero-based contiguous  Inputs=2  zeroidx=on
  Multiport Switch1 : MultiPortSwitch  DataPortOrder=Zero-based contiguous  Inputs=2  zeroidx=on
  Relational Operator : RelationalOperator  Operator===  OutDataTypeStr=boolean  RndMeth=Simplest
  Shift Arithmetic : ArithShift  BitShiftNumberSource=Input port  BitShiftNumber=8  BitShiftDirection=Left  DiagnosticForOORShift=Error
      settings: InputPortMap=u0,p1
  Shift Arithmetic1 : ArithShift  BitShiftNumberSource=Input port  BitShiftNumber=8  BitShiftDirection=Left  DiagnosticForOORShift=Error
      settings: InputPortMap=u0,p1
  Shift Arithmetic2 : ArithShift  BitShiftNumberSource=Input port  BitShiftNumber=8  BitShiftDirection=Right  DiagnosticForOORShift=Error
      settings: InputPortMap=u0,p1
  Signal Specification : SignalSpecification  OutDataTypeStr=fixdt(0, 36, 0)
  Vote : Constant  OutDataTypeStr=fixdt(0,1,0)  SampleTime=-1
  Zero : Constant  Value=0  OutDataTypeStr=fixdt(0,1,0)  SampleTime=-1
  hps : Outport
  wires:
  Block RAM/1(rd_data) -> Signal Specification/1
  Multiport Switch1/1 -> Shift Arithmetic2/1, Bitwise AND/2
  Signal Specification/1 -> Multiport Switch1/2
  Bitwise OR/1 -> Block RAM/1(wr_data), Delay5/1
  Bitwise AND/1 -> Bitwise OR/1
  Shift Arithmetic2/1 -> Bit Slice/1
  Add/1 -> Multiport Switch/3
  Multiport Switch/1 -> Bit Concat/2
  Bit Concat/1 -> Shift Arithmetic/1
  Shift Arithmetic/1 -> Bitwise OR/2
  Delay5/1 -> Multiport Switch1/3
  edge/1 -> Delay1/1
  address/1 -> Block RAM/4(rd_addr), Delay/1, Relational Operator/2
  mode/1 -> Multiport Switch/1
  shift/1 -> Delay4/1
  AND/1 -> Delay2/1
  Bit Slice/1 -> Add/2, hps/1
  Bitwise NOT/1 -> Bitwise AND/1
  Constant/1 -> Bit Concat/1
  Constant1/1 -> Shift Arithmetic1/1
  Delay/1 -> Block RAM/2(wr_addr), Relational Operator/1
  Delay1/1 -> Block RAM/3(wr_en), AND/1
  Delay2/1 -> Multiport Switch1/1
  Delay4/1 -> Shift Arithmetic2/2, Shift Arithmetic/2, Shift Arithmetic1/2
  Relational Operator/1 -> AND/2
  Shift Arithmetic1/1 -> Bitwise NOT/1
  Vote/1 -> Add/1
  Zero/1 -> Multiport Switch/2

== system gm_hybrid_lht/Hybrid LHT/Hybrid LHT Accumulator/Accumulator with Switches/Accumulator_instance18 ==
  shift : Inport  OutDataTypeStr=fixdt(0, 6, 0)  PortDimensions=1  SampleTime=8.33333333333333e-09
  mode : Inport  Port=2  OutDataTypeStr=boolean  PortDimensions=1  SampleTime=8.33333333333333e-09
  address : Inport  Port=3  OutDataTypeStr=fixdt(0, 11, 0)  PortDimensions=1  SampleTime=8.33333333333333e-09
  edge : Inport  Port=4  OutDataTypeStr=boolean  PortDimensions=1  SampleTime=8.33333333333333e-09
  AND : Logic  IconShape=distinctive  AllPortsSameDT=off  OutDataTypeStr=boolean
  Add : Sum  OutDataTypeStr=fixdt(0, ceil(log2(maxRho*2)), 0)
  Bit Concat : hdlsllib/Logic and Bit Operations/Bit Concat  numInputs=2
      settings: SourceProductName=Simulink
  Bit Slice : hdlsllib/Logic and Bit Operations/Bit Slice  lidx=voteWL-1  ridx=0
  Bitwise AND : simulink/Logic and Bit Operations/Bitwise Operator  logicop=AND  UseBitMask=off  NumInputPorts=2  BitMask=bin2dec('11011001')  BitMaskRealWorld=Stored Integer
  Bitwise NOT : simulink/Logic and Bit Operations/Bitwise Operator  logicop=NOT  UseBitMask=off  BitMask=bin2dec('11011001')  BitMaskRealWorld=Stored Integer
  Bitwise OR : simulink/Logic and Bit Operations/Bitwise Operator  logicop=OR  UseBitMask=off  NumInputPorts=2  BitMask=bin2dec('11011001')  BitMaskRealWorld=Stored Integer
  Block RAM : Subsystem
  Constant : Constant  Value=0  OutDataTypeStr=fixdt(0, 36-voteWL, 0)  SampleTime=-1
  Constant1 : Constant  Value=2^(voteWL)-1  OutDataTypeStr=fixdt(0, 36, 0)  SampleTime=-1
  Delay{,1..2,4..5} (5 alike) : Delay  DelayLength=1
  Multiport Switch : MultiPortSwitch  DataPortOrder=Zero-based contiguous  Inputs=2  zeroidx=on
  Multiport Switch1 : MultiPortSwitch  DataPortOrder=Zero-based contiguous  Inputs=2  zeroidx=on
  Relational Operator : RelationalOperator  Operator===  OutDataTypeStr=boolean  RndMeth=Simplest
  Shift Arithmetic : ArithShift  BitShiftNumberSource=Input port  BitShiftNumber=8  BitShiftDirection=Left  DiagnosticForOORShift=Error
      settings: InputPortMap=u0,p1
  Shift Arithmetic1 : ArithShift  BitShiftNumberSource=Input port  BitShiftNumber=8  BitShiftDirection=Left  DiagnosticForOORShift=Error
      settings: InputPortMap=u0,p1
  Shift Arithmetic2 : ArithShift  BitShiftNumberSource=Input port  BitShiftNumber=8  BitShiftDirection=Right  DiagnosticForOORShift=Error
      settings: InputPortMap=u0,p1
  Signal Specification : SignalSpecification  OutDataTypeStr=fixdt(0, 36, 0)
  Vote : Constant  OutDataTypeStr=fixdt(0,1,0)  SampleTime=-1
  Zero : Constant  Value=0  OutDataTypeStr=fixdt(0,1,0)  SampleTime=-1
  hps : Outport
  wires:
  Block RAM/1(rd_data) -> Signal Specification/1
  Multiport Switch1/1 -> Shift Arithmetic2/1, Bitwise AND/2
  Signal Specification/1 -> Multiport Switch1/2
  Bitwise OR/1 -> Block RAM/1(wr_data), Delay5/1
  Bitwise AND/1 -> Bitwise OR/1
  Shift Arithmetic2/1 -> Bit Slice/1
  Add/1 -> Multiport Switch/3
  Multiport Switch/1 -> Bit Concat/2
  Bit Concat/1 -> Shift Arithmetic/1
  Shift Arithmetic/1 -> Bitwise OR/2
  Delay5/1 -> Multiport Switch1/3
  edge/1 -> Delay1/1
  address/1 -> Block RAM/4(rd_addr), Delay/1, Relational Operator/2
  mode/1 -> Multiport Switch/1
  shift/1 -> Delay4/1
  AND/1 -> Delay2/1
  Bit Slice/1 -> Add/2, hps/1
  Bitwise NOT/1 -> Bitwise AND/1
  Constant/1 -> Bit Concat/1
  Constant1/1 -> Shift Arithmetic1/1
  Delay/1 -> Block RAM/2(wr_addr), Relational Operator/1
  Delay1/1 -> Block RAM/3(wr_en), AND/1
  Delay2/1 -> Multiport Switch1/1
  Delay4/1 -> Shift Arithmetic2/2, Shift Arithmetic/2, Shift Arithmetic1/2
  Relational Operator/1 -> AND/2
  Shift Arithmetic1/1 -> Bitwise NOT/1
  Vote/1 -> Add/1
  Zero/1 -> Multiport Switch/2

== system gm_hybrid_lht/Hybrid LHT/Hybrid LHT Accumulator/Accumulator with Switches/Accumulator_instance19 ==
  shift : Inport  OutDataTypeStr=fixdt(0, 6, 0)  PortDimensions=1  SampleTime=8.33333333333333e-09
  mode : Inport  Port=2  OutDataTypeStr=boolean  PortDimensions=1  SampleTime=8.33333333333333e-09
  address : Inport  Port=3  OutDataTypeStr=fixdt(0, 11, 0)  PortDimensions=1  SampleTime=8.33333333333333e-09
  edge : Inport  Port=4  OutDataTypeStr=boolean  PortDimensions=1  SampleTime=8.33333333333333e-09
  AND : Logic  IconShape=distinctive  AllPortsSameDT=off  OutDataTypeStr=boolean
  Add : Sum  OutDataTypeStr=fixdt(0, ceil(log2(maxRho*2)), 0)
  Bit Concat : hdlsllib/Logic and Bit Operations/Bit Concat  numInputs=2
      settings: SourceProductName=Simulink
  Bit Slice : hdlsllib/Logic and Bit Operations/Bit Slice  lidx=voteWL-1  ridx=0
  Bitwise AND : simulink/Logic and Bit Operations/Bitwise Operator  logicop=AND  UseBitMask=off  NumInputPorts=2  BitMask=bin2dec('11011001')  BitMaskRealWorld=Stored Integer
  Bitwise NOT : simulink/Logic and Bit Operations/Bitwise Operator  logicop=NOT  UseBitMask=off  BitMask=bin2dec('11011001')  BitMaskRealWorld=Stored Integer
  Bitwise OR : simulink/Logic and Bit Operations/Bitwise Operator  logicop=OR  UseBitMask=off  NumInputPorts=2  BitMask=bin2dec('11011001')  BitMaskRealWorld=Stored Integer
  Block RAM : Subsystem
  Constant : Constant  Value=0  OutDataTypeStr=fixdt(0, 36-voteWL, 0)  SampleTime=-1
  Constant1 : Constant  Value=2^(voteWL)-1  OutDataTypeStr=fixdt(0, 36, 0)  SampleTime=-1
  Delay{,1..2,4..5} (5 alike) : Delay  DelayLength=1
  Multiport Switch : MultiPortSwitch  DataPortOrder=Zero-based contiguous  Inputs=2  zeroidx=on
  Multiport Switch1 : MultiPortSwitch  DataPortOrder=Zero-based contiguous  Inputs=2  zeroidx=on
  Relational Operator : RelationalOperator  Operator===  OutDataTypeStr=boolean  RndMeth=Simplest
  Shift Arithmetic : ArithShift  BitShiftNumberSource=Input port  BitShiftNumber=8  BitShiftDirection=Left  DiagnosticForOORShift=Error
      settings: InputPortMap=u0,p1
  Shift Arithmetic1 : ArithShift  BitShiftNumberSource=Input port  BitShiftNumber=8  BitShiftDirection=Left  DiagnosticForOORShift=Error
      settings: InputPortMap=u0,p1
  Shift Arithmetic2 : ArithShift  BitShiftNumberSource=Input port  BitShiftNumber=8  BitShiftDirection=Right  DiagnosticForOORShift=Error
      settings: InputPortMap=u0,p1
  Signal Specification : SignalSpecification  OutDataTypeStr=fixdt(0, 36, 0)
  Vote : Constant  OutDataTypeStr=fixdt(0,1,0)  SampleTime=-1
  Zero : Constant  Value=0  OutDataTypeStr=fixdt(0,1,0)  SampleTime=-1
  hps : Outport
  wires:
  Block RAM/1(rd_data) -> Signal Specification/1
  Multiport Switch1/1 -> Shift Arithmetic2/1, Bitwise AND/2
  Signal Specification/1 -> Multiport Switch1/2
  Bitwise OR/1 -> Block RAM/1(wr_data), Delay5/1
  Bitwise AND/1 -> Bitwise OR/1
  Shift Arithmetic2/1 -> Bit Slice/1
  Add/1 -> Multiport Switch/3
  Multiport Switch/1 -> Bit Concat/2
  Bit Concat/1 -> Shift Arithmetic/1
  Shift Arithmetic/1 -> Bitwise OR/2
  Delay5/1 -> Multiport Switch1/3
  edge/1 -> Delay1/1
  address/1 -> Block RAM/4(rd_addr), Delay/1, Relational Operator/2
  mode/1 -> Multiport Switch/1
  shift/1 -> Delay4/1
  AND/1 -> Delay2/1
  Bit Slice/1 -> Add/2, hps/1
  Bitwise NOT/1 -> Bitwise AND/1
  Constant/1 -> Bit Concat/1
  Constant1/1 -> Shift Arithmetic1/1
  Delay/1 -> Block RAM/2(wr_addr), Relational Operator/1
  Delay1/1 -> Block RAM/3(wr_en), AND/1
  Delay2/1 -> Multiport Switch1/1
  Delay4/1 -> Shift Arithmetic2/2, Shift Arithmetic/2, Shift Arithmetic1/2
  Relational Operator/1 -> AND/2
  Shift Arithmetic1/1 -> Bitwise NOT/1
  Vote/1 -> Add/1
  Zero/1 -> Multiport Switch/2

== system gm_hybrid_lht/Hybrid LHT/Hybrid LHT Accumulator/Accumulator with Switches/Accumulator_instance2 ==
  shift : Inport  OutDataTypeStr=fixdt(0, 6, 0)  PortDimensions=1  SampleTime=8.33333333333333e-09
  mode : Inport  Port=2  OutDataTypeStr=boolean  PortDimensions=1  SampleTime=8.33333333333333e-09
  address : Inport  Port=3  OutDataTypeStr=fixdt(0, 11, 0)  PortDimensions=1  SampleTime=8.33333333333333e-09
  edge : Inport  Port=4  OutDataTypeStr=boolean  PortDimensions=1  SampleTime=8.33333333333333e-09
  AND : Logic  IconShape=distinctive  AllPortsSameDT=off  OutDataTypeStr=boolean
  Add : Sum  OutDataTypeStr=fixdt(0, ceil(log2(maxRho*2)), 0)
  Bit Concat : hdlsllib/Logic and Bit Operations/Bit Concat  numInputs=2
      settings: SourceProductName=Simulink
  Bit Slice : hdlsllib/Logic and Bit Operations/Bit Slice  lidx=voteWL-1  ridx=0
  Bitwise AND : simulink/Logic and Bit Operations/Bitwise Operator  logicop=AND  UseBitMask=off  NumInputPorts=2  BitMask=bin2dec('11011001')  BitMaskRealWorld=Stored Integer
  Bitwise NOT : simulink/Logic and Bit Operations/Bitwise Operator  logicop=NOT  UseBitMask=off  BitMask=bin2dec('11011001')  BitMaskRealWorld=Stored Integer
  Bitwise OR : simulink/Logic and Bit Operations/Bitwise Operator  logicop=OR  UseBitMask=off  NumInputPorts=2  BitMask=bin2dec('11011001')  BitMaskRealWorld=Stored Integer
  Block RAM : Subsystem
  Constant : Constant  Value=0  OutDataTypeStr=fixdt(0, 36-voteWL, 0)  SampleTime=-1
  Constant1 : Constant  Value=2^(voteWL)-1  OutDataTypeStr=fixdt(0, 36, 0)  SampleTime=-1
  Delay{,1..2,4..5} (5 alike) : Delay  DelayLength=1
  Multiport Switch : MultiPortSwitch  DataPortOrder=Zero-based contiguous  Inputs=2  zeroidx=on
  Multiport Switch1 : MultiPortSwitch  DataPortOrder=Zero-based contiguous  Inputs=2  zeroidx=on
  Relational Operator : RelationalOperator  Operator===  OutDataTypeStr=boolean  RndMeth=Simplest
  Shift Arithmetic : ArithShift  BitShiftNumberSource=Input port  BitShiftNumber=8  BitShiftDirection=Left  DiagnosticForOORShift=Error
      settings: InputPortMap=u0,p1
  Shift Arithmetic1 : ArithShift  BitShiftNumberSource=Input port  BitShiftNumber=8  BitShiftDirection=Left  DiagnosticForOORShift=Error
      settings: InputPortMap=u0,p1
  Shift Arithmetic2 : ArithShift  BitShiftNumberSource=Input port  BitShiftNumber=8  BitShiftDirection=Right  DiagnosticForOORShift=Error
      settings: InputPortMap=u0,p1
  Signal Specification : SignalSpecification  OutDataTypeStr=fixdt(0, 36, 0)
  Vote : Constant  OutDataTypeStr=fixdt(0,1,0)  SampleTime=-1
  Zero : Constant  Value=0  OutDataTypeStr=fixdt(0,1,0)  SampleTime=-1
  hps : Outport
  wires:
  Block RAM/1(rd_data) -> Signal Specification/1
  Multiport Switch1/1 -> Shift Arithmetic2/1, Bitwise AND/2
  Signal Specification/1 -> Multiport Switch1/2
  Bitwise OR/1 -> Block RAM/1(wr_data), Delay5/1
  Bitwise AND/1 -> Bitwise OR/1
  Shift Arithmetic2/1 -> Bit Slice/1
  Add/1 -> Multiport Switch/3
  Multiport Switch/1 -> Bit Concat/2
  Bit Concat/1 -> Shift Arithmetic/1
  Shift Arithmetic/1 -> Bitwise OR/2
  Delay5/1 -> Multiport Switch1/3
  edge/1 -> Delay1/1
  address/1 -> Block RAM/4(rd_addr), Delay/1, Relational Operator/2
  mode/1 -> Multiport Switch/1
  shift/1 -> Delay4/1
  AND/1 -> Delay2/1
  Bit Slice/1 -> Add/2, hps/1
  Bitwise NOT/1 -> Bitwise AND/1
  Constant/1 -> Bit Concat/1
  Constant1/1 -> Shift Arithmetic1/1
  Delay/1 -> Block RAM/2(wr_addr), Relational Operator/1
  Delay1/1 -> Block RAM/3(wr_en), AND/1
  Delay2/1 -> Multiport Switch1/1
  Delay4/1 -> Shift Arithmetic2/2, Shift Arithmetic/2, Shift Arithmetic1/2
  Relational Operator/1 -> AND/2
  Shift Arithmetic1/1 -> Bitwise NOT/1
  Vote/1 -> Add/1
  Zero/1 -> Multiport Switch/2
